simulink model "Vehicle_Model_Controller_Mar18"  (R2020b)
settings: Solver=VariableStepAuto  StartTime=0.0  StopTime=20  FixedStep=0.015  MaxStep=0.015  RelTol=1e-3
model workspace (MAT data in the model file):
  Kp = 10
  understeer_gradient = 0.05
values from neighbouring files (symbols this model uses):
  a = Simulink.Parameter(1.14)    [startup.m]
  A1 = Simulink.Parameter(39.8344)    [startup.m]
  A2 = Simulink.Parameter(813.0780)    [startup.m]
  b = Simulink.Parameter(-0.03291)    [startup.m]
  B1 = Simulink.Parameter(0.000001287)    [startup.m]
  B2 = Simulink.Parameter(-0.002325)    [startup.m]
  B3 = Simulink.Parameter(3.797)    [startup.m]
  brakecoeff = Simulink.Parameter([((1.23*25.4/2)^2 * pi * 2) * (0.4) * (0.1), ((1*25.4/2)^2 * pi * 2) * (0.4) * (0.1)])    [startup.m]
  c = Simulink.Parameter(-1.14)    [startup.m]
  C1 = Simulink.Parameter(-0.000000002541)    [startup.m]
  C2 = Simulink.Parameter(0.000005279)    [startup.m]
  C3 = Simulink.Parameter(-0.003943)    [startup.m]
  C4 = Simulink.Parameter(3.634)    [startup.m]
  C_param = Simulink.Parameter([0 13757.41 21278.97 26666.02 30253.47 30313.18 30313.18])    [startup.m]
  d = Simulink.Parameter(-1.027)    [startup.m]
  driver_gain = 1    [startup.m]
  FZ_C = Simulink.Parameter([0 204.13 427.04 668.1 895.72 1124.40 1324.40])    [startup.m]
  g = Simulink.Parameter(9.81)    [startup.m]
  gearbox_efficiency = Simulink.Parameter([0.97 0.97 0.97 0.97])    [startup.m]
  gr = Simulink.Parameter([6.63043, 6.63043, 7.95652, 7.95652])    [startup.m]
  I = 30    [startup.m]
  inch2mm = Simulink.Parameter(25.4)    [startup.m]
  J_z = Simulink.Parameter(75)    [startup.m]
  k_limit = Simulink.Parameter(3.461)    [startup.m]
  Ku = Simulink.Parameter(0.24 / g.Value)    [startup.m]
  l = Simulink.Parameter([0.7922471, 0.7828529])    [startup.m]
  max_yaw_field = Simulink.Parameter([1.34 1.34 1.34 1.66 1.14 1.24 0.754 0.849 0.85 0.85])    [startup.m]
  mech_brake = Simulink.Parameter(-0.5)    [startup.m]
  min_speed_regen = Simulink.Parameter(85)    [startup.m]
  motor_efficiency = Simulink.Parameter([0.85, 0.85, 0.85, 0.85])    [startup.m]
  motor_limit_power = Simulink.Parameter([15000, 15000, 15000, 15000])    [startup.m]
  motor_limit_torque = Simulink.Parameter([-25, 25])    [startup.m]
  mu_factor = Simulink.Parameter(2/3)    [startup.m]
  P = 30    [startup.m]
  ramp_rate = 1    [startup.m]
  RE = Simulink.Parameter(0.2228169203)    [startup.m]
  s = Simulink.Parameter([0.647895, 0.62102])    [startup.m]
  S1 = Simulink.Parameter(-7 * (10^(-5)))    [startup.m]
  S2 = Simulink.Parameter(0.0038)    [startup.m]
  S3 = Simulink.Parameter(-0.6535)    [startup.m]
  S4 = Simulink.Parameter(-0.1061)    [startup.m]
  steer_slope = Simulink.Parameter(0.00962)    [startup.m]
  steering_freq = pi    (= 3.14159265359)    [startup.m]
  T = 100    [startup.m]
  T2F = Simulink.Parameter(single([29 29 35 35]))    [startup.m]
  tau = Simulink.Parameter(0)    [startup.m]
  time_delay = 0.022    [startup.m]
  V_target = Simulink.Parameter([0 3 6 9 12 15 18 21 25 31])    [startup.m]
undefined symbols (not defined in the file or in its folder): DiscIntNeverNeededParam
libraries: fl_lib x32, nesl_utility x24, sdl_lib x8, pid_lib x1, autolibshared x1, autolibdatasheetbattery x1
(part 3 of 3)

== matlab function Vehicle_Model_Controller_Mar18/Motor and Battery/Motors/   ==
  data: Battery_Voltage input; ang_vel_RAD input; battery_current output; Motor_torque input; battery_power output
function [battery_current, battery_power]= get_batt_curr(Battery_Voltage, ang_vel_RAD, Motor_torque)
%% Current Draw
% Developers:    Demetrius Gulewicz

% Developed for: Purdue Electric Racing
% Date:          09/18/2021
%
% Definitions:
% ang_vel_RAD:   Angular velocity of each wheel on the wheel fixed y axis [RAD]
% Motor_torque:  Torque the motor actually outputs                 [Ncm]
% Battery_Voltage: The voltage of the battery                      [V]

%% Definitions
a = 0.0411;
b = 2.7976;
c = 45.978;

t = Motor_torque;
w = ang_vel_RAD;
v = Battery_Voltage;

e = 85;

%% Calculate Current Draw
%x0 = [20, 20, 20, 20];
%options = optimoptions('fsolve','Algorithm','Levenberg-Marquardt');
%F = @(x) ([(a * x(1)^3) + (b * x(1)^2) + (c * x(1)), ] .* v) - (t .* w);
%battery_current = sum(fsolve(F,x0,options));

battery_current = sum((t .* w) ./ (e .* v));
battery_power = battery_current * Battery_Voltage;
end
